simulink model "PitchSysold"  (R2019b)
settings: Solver=ode1  StartTime=0.00  StopTime=10.00  FixedStep=0.01  RelTol=1e-3  EnableMultiTasking=on
values from neighbouring files (symbols this model uses):
  Jp = 2*m1*(l2^2)    (= 0.0004949)    [heli.m]
  k_d = 1.5    [heli.m]
  k_s = 4    [heli.m]
  l2 = 0.070    (= 0.07)    [heli.m]
settings Model: Creator=bjones  LastModifiedBy=seb
settings DataIOCC: SaveFormat=Array  SignalLoggingSaveFormat=ModelDataLogs  ReturnWorkspaceOutputs=off
settings OptimizationCC: BlockReduction=off  BooleanDataType=off  ExpressionDepthLimit=2147483647  LifeSpan=inf
settings DebuggingCC: SaveWithParameterizedLinksMsg=none  UnderspecifiedInitializationDetection=Classic  MergeDetectMultiDrivingBlocksExec=none  SignalResolutionControl=TryResolveAllWithWarning  MultiTaskDSMMsg=warning  MultiTaskCondExecSysMsg=none  FcnCallInpInsideContextMsg=warning  StateNameClashWarn=warning  SFUnexpectedBacktrackingDiag=warning  SFNoUnconditionalDefaultTransitionDiag=warning  SFExecutionAtInitializationDiag=none  ArithmeticOperatorsInVariantConditions=warning
settings HardwareCC: ProdBitPerPointer=32  ProdBitPerSizeT=32  ProdBitPerPtrDiffT=32  ProdLargestAtomicFloat=None  ProdIntDivRoundTo=Undefined  ProdEndianess=Unspecified  ProdWordSize=32  ProdHWDeviceType=32-bit Generic  TargetUnknown=on
settings ModelReferenceCC: PropagateSignalLabelsOutOfModel=off
settings SFSimCC: SimUseLocalCustomCode=off  CustomCodeUndefinedFunction=UseInterfaceOnly
settings RTWCC: RTWUseLocalCustomCode=off
settings CodeAppCC: StateflowObjectComments=on
settings GRTTargetCC: TargetLangStandard=C89/C90 (ANSI)  CombineOutputUpdateFcns=off  GRTInterface=on
settings ConfigComp: CovMetricSettings=dw  CovSaveCumulativeToWorkspaceVar=on  CovSaveSingleToWorkspaceVar=on  CovExternalEMLEnable=off  CovSFcnEnable=off

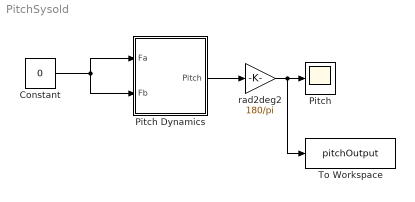
== system PitchSysold ==
  Constant : Constant  Value=0
  Pitch : Scope
  Pitch Dynamics : Subsystem
  To Workspace : ToWorkspace  VariableName=pitchOutput  SaveFormat=Timeseries  SampleTime=-1
  rad2deg2 : Gain  Gain=180/pi  SaturateOnIntegerOverflow=on  OutDataTypeStr=Inherit: Same as input  ParamDataTypeStr=Inherit: Same as input
  wires:
  Pitch Dynamics/1(Pitch) -> rad2deg2/1
  rad2deg2/1 -> To Workspace/1, Pitch/1
  Constant/1 -> Pitch Dynamics/1(Fa), Pitch Dynamics/2(Fb)

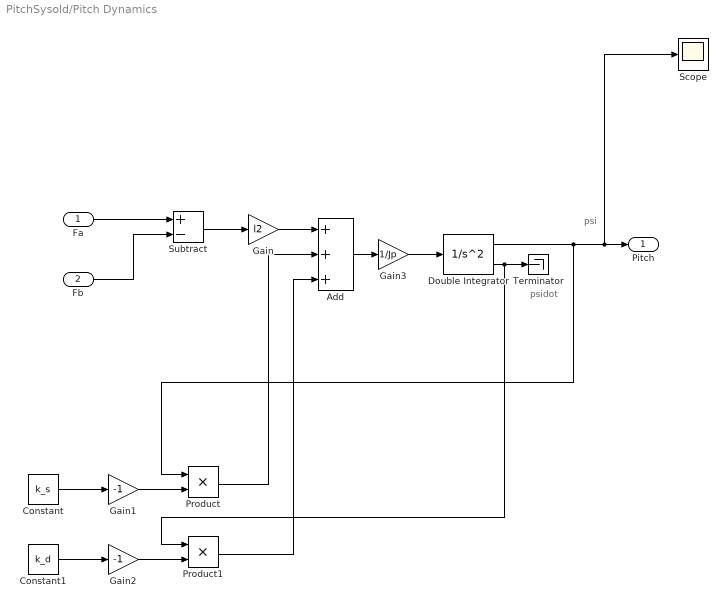
== system PitchSysold/Pitch Dynamics ==
  note: psi
  note: psidot
  Fa : Inport
  Fb : Inport  Port=2
  Add : Sum  Inputs=+++
  Constant : Constant  Value=k_s
  Constant1 : Constant  Value=k_d
  Double Integrator : SecondOrderIntegrator  ICX=p_lim_u  LimitX=on  UpperLimitX=p_lim_u  LowerLimitX=p_lim_l
  Gain : Gain  Gain=l2
  Gain1 : Gain  Gain=-1
  Gain2 : Gain  Gain=-1
  Gain3 : Gain  Gain=1/Jp
  Product : Product
  Product1 : Product
  Scope : Scope
  Subtract : Sum  Inputs=+-
  Terminator : Terminator
  Pitch : Outport
  wires:
  Double Integrator/1 -> Product/1, Scope/1, Pitch/1
  Double Integrator/2 -> Product1/1, Terminator/1
  Fa/1 -> Subtract/1
  Fb/1 -> Subtract/2
  Subtract/1 -> Gain/1
  Gain/1 -> Add/1
  Gain1/1 -> Product/2
  Gain2/1 -> Product1/2
  Product/1 -> Add/2
  Product1/1 -> Add/3
  Constant/1 -> Gain1/1
  Constant1/1 -> Gain2/1
  Add/1 -> Gain3/1
  Gain3/1 -> Double Integrator/1
